simulink model "final"  (R2015a)
settings: Solver=FixedStepDiscrete  SolverMode=SingleTasking  StartTime=0.0  StopTime=3  RelTol=1e-3
PreLoadFcn:
  | Ts_Power=1e-6
  | Ts_Control=100e-6
values from neighbouring files (symbols this model uses):
  Iph_array = Iph*Npar    (= 29.801)    [sunpower305.m]
  Isat_array = Isat*Npar    (= 5.8765e-08)    [sunpower305.m]
  Rp_array = Rp*Nser/Npar    (= 198.702)    [sunpower305.m]
  Rs_array = Rs*Nser/Npar    (= 0.0075996)    [sunpower305.m]
  Ts = Ts_Power    (= 1e-06)    [sunpower305.m]
  VT_array = VT*Nser    (= 3.20466023218)    [sunpower305.m]
undefined symbols (not defined in the file or in its folder): D1, Delta, level, sigbuilder_block
libraries: powerlib x29, powerlib_extras x6, simulink x4
(part 2 of 2)

== system final/VSC Control/VDC Regulator ==
  Vdc_mes : Inport  PortDimensions=1
  Vdc_ref : Inport  Port=2  PortDimensions=1
  PI : simulink/Continuous/PID Controller  Controller=PI  TimeDomain=Discrete-time  SampleTime=Ts  IntegratorMethod=Trapezoidal  FilterMethod=Forward Euler  Form=Parallel  UseFilter=on  ControllerParametersSource=internal  P=Kp_VDCreg  I=Ki_VDCreg  D=0  N=100  InitialConditionSource=internal  InitialConditionForIntegrator=0  InitialConditionForFilter=0  ExternalReset=none  LimitOutput=on  UpperSaturationLimit=1.5  LowerSaturationLimit=-1.5  LinearizeAsGain=off  AntiWindupMode=none  Kb=1  TrackingMode=off  Kt=1  PParamMin=[]  PParamMax=[]  IParamMin=[]  IParamMax=[]  DParamMin=[]  DParamMax=[]  NParamMin=[]  NParamMax=[]  KbParamMin=[]  KbParamMax=[]  KtParamMin=[]  KtParamMax=[]  POutMin=[]  POutMax=[]  IOutMin=[]  IOutMax=[]  DOutMin=[]  DOutMax=[]  NOutMin=[]  NOutMax=[]  KbOutMin=[]  KbOutMax=[]  KtOutMin=[]  KtOutMax=[]  IntegratorOutMin=[]  IntegratorOutMax=[]  FilterOutMin=[]  FilterOutMax=[]  SumOutMin=[]  SumOutMax=[]  SumI1OutMin=[]  SumI1OutMax=[]  SumI2OutMin=[]  SumI2OutMax=[]  SumI3OutMin=[]  SumI3OutMax=[]  SumDOutMin=[]  SumDOutMax=[]  SaturationOutMin=[]  SaturationOutMax=[]  IntegratorContinuousStateAttributes=''  IntegratorStateMustResolveToSignalObject=off  IntegratorRTWStateStorageClass=Auto  FilterContinuousStateAttributes=''  FilterStateMustResolveToSignalObject=off  FilterRTWStateStorageClass=Auto  DifferentiatorICPrevScaledInput=0  DifferentiatorOutMin=[]  DifferentiatorOutMax=[]
  Rtot_pu3 : Gain  Gain=1/Vnom_dc  SaturateOnIntegerOverflow=on  OutDataTypeStr=Inherit: Same as input  ParamDataTypeStr=Inherit: Same as input
  Sum : Sum  Inputs=|+-
  Id_ref : Outport  SampleTime=Ts  InitialOutput=0
  wires:
  Sum/1 -> Rtot_pu3/1
  Vdc_mes/1 -> Sum/1
  Vdc_ref/1 -> Sum/2
  Rtot_pu3/1 -> PI/1
  PI/1 -> Id_ref/1
